simulink model "MPC_Guido_v1_2020a"  (R2020a)
settings: Solver=FixedStepAuto  StartTime=0.0  StopTime=21  RelTol=1e-3
undefined symbols (not defined in the file): Bvx, Bvy, Bw, C, Cvx, Cvy, Cw, D, d, DiscIntNeverNeededParam, Gam, J, K_fsfb, K_int, Kt, l, M, Phi, r, Ti, Ts
libraries: mpclib x3, simulink x1
settings Model: Creator=User  LastModifiedBy=User
settings SolverCC: ZeroCrossControl=EnableAll  ZeroCrossAlgorithm=Adaptive
settings DebuggingCC: IgnoredZcDiagnostic=none

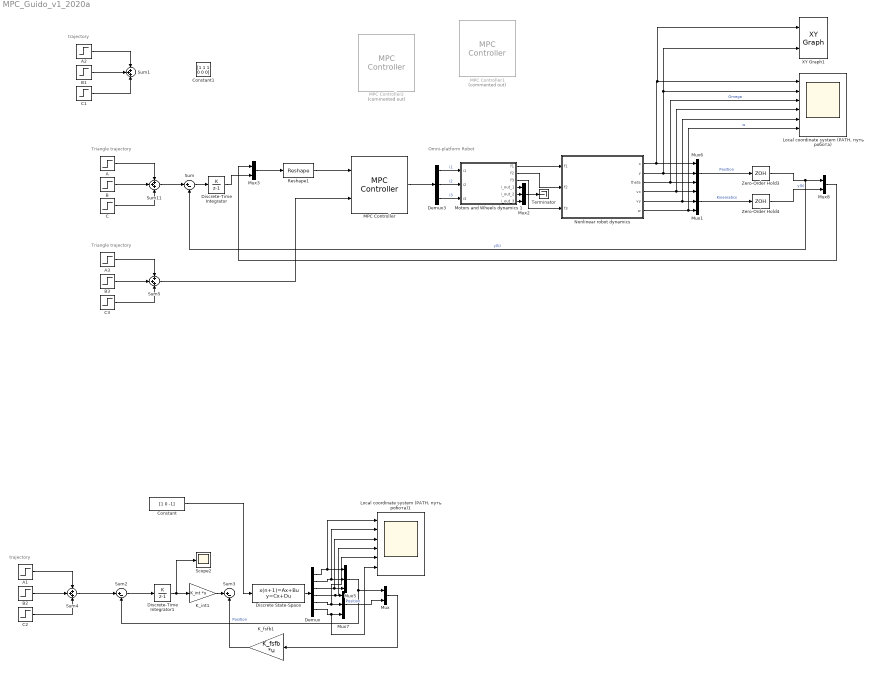
== system MPC_Guido_v1_2020a ==
  note: Omni-platform Robot
  note: Triangle trajectory
  note: trajectory
  note: trajectory
  note: Triangle trajectory
  A : Step  Time=0  Before=[1 0.5 pi/2]  After=[0.5 -sqrt(3)/2 1]  SampleTime=Ts
  A1 : Step  Time=0  Before=[0 0 0]  After=[1 1 0]  SampleTime=Ts
  A2 : Step  Time=0  Before=[0 0 0]  After=[1 1 0]  SampleTime=Ts
  A3 : Step  Time=0  Before=[1 0.5 pi/2 0 0 0 0 0 0]  After=[0.5 -sqrt(3)/2 1 0 0 0 0 0 0]  SampleTime=Ts
  B : Step  Time=7  Before=[0 0 0]  After=[-1 0 1]  SampleTime=Ts
  B1 : Step  Time=6  Before=[0 0 0]  After=[0 0 pi]  SampleTime=Ts
  B2 : Step  Time=6  Before=[0 0 0]  After=[0 0 pi]  SampleTime=Ts
  B3 : Step  Time=7  Before=[0 0 0 0 0 0 0 0 0]  After=[-1 0 1 0 0 0 0 0 0]  SampleTime=Ts
  C : Step  Time=14  Before=[0 0 0]  After=[0.5 sqrt(3)/2 0]  SampleTime=Ts
  C1 : Step  Time=12  Before=[0 0 0]  After=[1 1 0]  SampleTime=Ts
  C2 : Step  Time=12  Before=[0 0 0]  After=[1 1 0]  SampleTime=Ts
  C3 : Step  Time=14  Before=[0 0 0 0 0 0 0 0 0]  After=[0.5 sqrt(3)/2 0 0 0 0 0 0 0]  SampleTime=Ts
  Constant : Constant  Value=[1 0 -1]  SampleTime=Ts
  Constant1 : Constant  Value=[1 1 1 0 0 0]  SampleTime=Ts
  Demux : Demux  Outputs=6
  Demux3 : Demux  Outputs=3
  Discrete State-Space : DiscreteStateSpace  A=Phi  B=Gam  C=C  D=D  SampleTime=Ts
  Discrete-Time Integrator : DiscreteIntegrator  IntegratorMethod=Accumulation: Forward Euler  SampleTime=-1  ICPrevOutput=DiscIntNeverNeededParam  ICPrevScaledInput=DiscIntNeverNeededParam
  Discrete-Time Integrator1 : DiscreteIntegrator  IntegratorMethod=Accumulation: Forward Euler  InitialCondition=[ 0 0 0]  SampleTime=Ts  ICPrevOutput=DiscIntNeverNeededParam  ICPrevScaledInput=DiscIntNeverNeededParam
  K_fsfb1 : Gain  Gain=K_fsfb  Multiplication=Matrix(K*u) (u vector)
  K_int1 : Gain  Gain=K_int  Multiplication=Matrix(K*u) (u vector)
  "Local coordinate system (PATH, путь робота)" : Scope  NumInputPorts=6
  "Local coordinate system (PATH, путь робота)1" : Scope  NumInputPorts=6
  MPC Controller : mpclib/MPC Controller  SCDEnableBlockLinearizationSpecification=on  mpcobj=mpc1  is_multiple=0  enable_value=0  return_u0=off  updateMPCinCallerWorkspace=on  md_inport=off  mv_inport=off  uref_inport=off  return_cost=off  return_mvseq=off  return_qpstatus=off  return_xseq=off  return_state=off  return_ovseq=off  state_inport=off  umin_inport=off  umax_inport=off  ymin_inport=off  ymax_inport=off  cc_inport=off  ywt_inport=off  uwt_inport=off  duwt_inport=off  rhoeps_inport=off  pm_inport=off  MaximumP=10  HorizonChoice=FixedHorizon  n_ts=0.1  n_p=20  n_mv=3  n_md=0  n_ud=0  n_mo=9  n_uo=0  BlockDataType=double  SampleTimeInherited=off  switch_inport=off
  MPC Controller1 : mpclib/MPC Controller  Commented=on  SCDEnableBlockLinearizationSpecification=on  is_multiple=0  enable_value=0  return_u0=off  updateMPCinCallerWorkspace=on  md_inport=off  mv_inport=off  uref_inport=off  return_cost=off  return_mvseq=off  return_qpstatus=off  return_xseq=off  return_state=off  return_ovseq=off  state_inport=off  umin_inport=off  umax_inport=off  ymin_inport=off  ymax_inport=off  cc_inport=off  ywt_inport=off  uwt_inport=off  duwt_inport=off  rhoeps_inport=off  pm_inport=off  MaximumP=10  HorizonChoice=FixedHorizon  n_ts=0.02  n_p=100  n_mv=3  n_md=0  n_ud=0  n_mo=6  n_uo=0  BlockDataType=double  SampleTimeInherited=off  switch_inport=off
  MPC Controller2 : mpclib/MPC Controller  Commented=on  SCDEnableBlockLinearizationSpecification=on  is_multiple=0  enable_value=0  return_u0=off  updateMPCinCallerWorkspace=on  md_inport=off  mv_inport=off  uref_inport=off  return_cost=off  return_mvseq=off  return_qpstatus=off  return_xseq=off  return_state=off  return_ovseq=off  state_inport=off  umin_inport=off  umax_inport=off  ymin_inport=off  ymax_inport=off  cc_inport=off  ywt_inport=off  uwt_inport=off  duwt_inport=off  rhoeps_inport=off  pm_inport=off  MaximumP=10  HorizonChoice=FixedHorizon  n_ts=0.05  n_p=30  n_mv=3  n_md=0  n_ud=0  n_mo=6  n_uo=0  BlockDataType=double  SampleTimeInherited=off  switch_inport=off
  Motors and Wheels dynamics 1 : Subsystem
  Mux : Mux  Inputs=2
  Mux{1..2,5..7} (5 alike) : Mux  Inputs=3
  Mux3 : Mux  Inputs=2
  Mux8 : Mux  Inputs=2
  Nonlinear robot dynamics : Subsystem
  Reshape1 : Reshape  OutputDimensionality=Customize  OutputDimensions=[9,1]
  Scope2 : Scope
  Sum : Sum  Inputs=|+-
  Sum{1,4..5,11} (4 alike) : Sum  Inputs=+++
  Sum2 : Sum  Inputs=|+-
  Sum3 : Sum  Inputs=|+-
  Terminator : Terminator
  XY Graph1 : simulink/Sinks/XY Graph  xmin=-1  xmax=1  ymin=-1  ymax=1  st=-1
  Zero-Order Hold3 : ZeroOrderHold  SampleTime=0.05
  Zero-Order Hold4 : ZeroOrderHold  SampleTime=0.05
  wires:
  Nonlinear robot dynamics/1(x) -> XY Graph1/1, "Local coordinate system (PATH, путь робота)"/1, Mux6/1
  Nonlinear robot dynamics/2(y) -> XY Graph1/2, "Local coordinate system (PATH, путь робота)"/2, Mux6/2
  Nonlinear robot dynamics/3(theta) -> "Local coordinate system (PATH, путь робота)"/3, Mux6/3  "Omega"
  Mux6/1 -> Zero-Order Hold3/1  "Position"
  C/1 -> Sum11/3
  Zero-Order Hold3/1 -> Mux8/1, Sum/2  "y(k)"
  A/1 -> Sum11/1
  B/1 -> Sum11/2
  Nonlinear robot dynamics/5(vy) -> Mux1/2, "Local coordinate system (PATH, путь робота)"/5
  Nonlinear robot dynamics/6(w) -> Mux1/3, "Local coordinate system (PATH, путь робота)"/6  "w"
  Nonlinear robot dynamics/4(vx) -> Mux1/1, "Local coordinate system (PATH, путь робота)"/4
  Demux3/1 -> Motors and Wheels dynamics 1/1(i1)  "i1"
  Demux3/2 -> Motors and Wheels dynamics 1/2(i2)  "i2"
  Demux3/3 -> Motors and Wheels dynamics 1/3(i3)  "i3"
  Zero-Order Hold4/1 -> Mux8/2  "y(k)"
  Mux1/1 -> Zero-Order Hold4/1  "Kinematics"
  C1/1 -> Sum1/3
  A2/1 -> Sum1/1
  B1/1 -> Sum1/2
  K_int1/1 -> Sum3/1
  Sum2/1 -> Discrete-Time Integrator1/1
  Discrete-Time Integrator1/1 -> Scope2/1, K_int1/1
  Discrete State-Space/1 -> Demux/1
  C2/1 -> Sum4/3
  Sum4/1 -> Sum2/1
  A1/1 -> Sum4/1
  B2/1 -> Sum4/2
  Demux/1 -> "Local coordinate system (PATH, путь робота)1"/1, Mux5/1
  Demux/2 -> "Local coordinate system (PATH, путь робота)1"/2, Mux5/2
  Demux/3 -> "Local coordinate system (PATH, путь робота)1"/3, Mux5/3
  Demux/4 -> "Local coordinate system (PATH, путь робота)1"/4, Mux7/1
  Demux/5 -> "Local coordinate system (PATH, путь робота)1"/5, Mux7/2
  Demux/6 -> "Local coordinate system (PATH, путь робота)1"/6, Mux7/3
  Mux5/1 -> Mux/1, Sum2/2  "Position"
  K_fsfb1/1 -> Sum3/2
  Mux7/1 -> Mux/2  "Position"
  Mux/1 -> K_fsfb1/1
  Constant/1 -> Discrete State-Space/1
  Motors and Wheels dynamics 1/1(f1) -> Nonlinear robot dynamics/1(f1)
  Motors and Wheels dynamics 1/2(f2) -> Nonlinear robot dynamics/2(f2)
  Motors and Wheels dynamics 1/3(f3) -> Nonlinear robot dynamics/3(f3)
  Motors and Wheels dynamics 1/4(i_out_1) -> Mux2/1
  Motors and Wheels dynamics 1/5(i_out_2) -> Mux2/2
  Motors and Wheels dynamics 1/6(i_out_3) -> Mux2/3
  Mux2/1 -> Terminator/1
  MPC Controller/1 -> Demux3/1
  Sum/1 -> Discrete-Time Integrator/1
  Sum11/1 -> Sum/1
  Mux3/1 -> Reshape1/1
  Mux8/1 -> Mux3/1
  Reshape1/1 -> MPC Controller/1
  Discrete-Time Integrator/1 -> Mux3/2
  Sum5/1 -> MPC Controller/2
  B3/1 -> Sum5/2
  A3/1 -> Sum5/1
  C3/1 -> Sum5/3

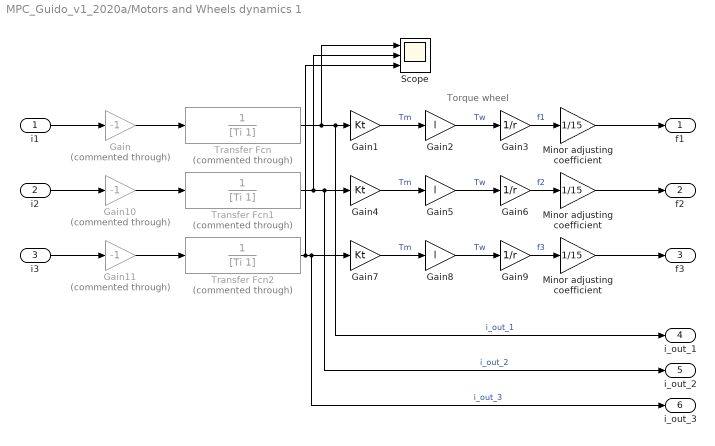
== system MPC_Guido_v1_2020a/Motors and Wheels dynamics 1 ==
  note: Torque wheel
  i1 : Inport
  i2 : Inport  Port=2
  i3 : Inport  Port=3
  Gain : Gain  Commented=through  Gain=-1
  Gain1 : Gain  Gain=Kt
  Gain10 : Gain  Commented=through  Gain=-1
  Gain11 : Gain  Commented=through  Gain=-1
  Gain2 : Gain  Gain=l
  Gain3 : Gain  Gain=1/r
  Gain4 : Gain  Gain=Kt
  Gain5 : Gain  Gain=l
  Gain6 : Gain  Gain=1/r
  Gain7 : Gain  Gain=Kt
  Gain8 : Gain  Gain=l
  Gain9 : Gain  Gain=1/r
  "Minor adjusting coefficient  " : Gain  Gain=1/15
  "Minor adjusting coefficient   " : Gain  Gain=1/15
  "Minor adjusting coefficient    " : Gain  Gain=1/15
  Scope : Scope  NumInputPorts=3
  Transfer Fcn : TransferFcn  Commented=through  Denominator=[Ti 1]  ContinuousStateAttributes='i_out_1'
  Transfer Fcn1 : TransferFcn  Commented=through  Denominator=[Ti 1]  ContinuousStateAttributes='i_out_2'
  Transfer Fcn2 : TransferFcn  Commented=through  Denominator=[Ti 1]  ContinuousStateAttributes='i_out_3'
  f1 : Outport
  f2 : Outport  Port=2
  f3 : Outport  Port=3
  i_out_1 : Outport  Port=4
  i_out_2 : Outport  Port=5
  i_out_3 : Outport  Port=6
  wires:
  i2/1 -> Gain10/1
  Gain1/1 -> Gain2/1  "Tm"
  Gain8/1 -> Gain9/1  "Tw"
  Gain5/1 -> Gain6/1  "Tw"
  Transfer Fcn/1 -> Scope/1, i_out_1/1, Gain1/1  "i_out_1"
  Transfer Fcn2/1 -> Scope/3, i_out_3/1, Gain7/1  "i_out_3"
  i3/1 -> Gain11/1
  Gain2/1 -> Gain3/1  "Tw"
  Gain7/1 -> Gain8/1  "Tm"
  Transfer Fcn1/1 -> Scope/2, i_out_2/1, Gain4/1  "i_out_2"
  Gain4/1 -> Gain5/1  "Tm"
  Gain3/1 -> "Minor adjusting coefficient  "/1  "f1"
  Gain6/1 -> "Minor adjusting coefficient   "/1  "f2"
  i1/1 -> Gain/1
  Gain9/1 -> "Minor adjusting coefficient    "/1  "f3"
  Gain/1 -> Transfer Fcn/1
  Gain10/1 -> Transfer Fcn1/1
  Gain11/1 -> Transfer Fcn2/1
  "Minor adjusting coefficient  "/1 -> f1/1
  "Minor adjusting coefficient   "/1 -> f2/1
  "Minor adjusting coefficient    "/1 -> f3/1

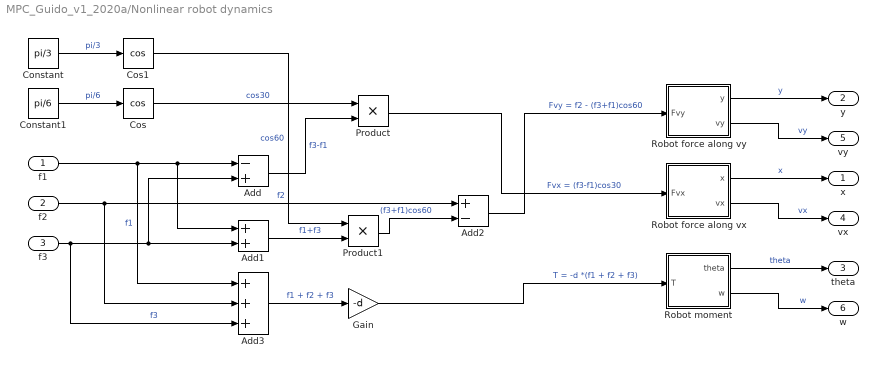
== system MPC_Guido_v1_2020a/Nonlinear robot dynamics ==
  f1 : Inport
  f2 : Inport  Port=2
  f3 : Inport  Port=3
  Add : Sum  Inputs=-+
  Add1 : Sum
  Add2 : Sum  Inputs=+-
  Add3 : Sum  Inputs=+++
  Constant : Constant  Value=pi/3
  Constant1 : Constant  Value=pi/6
  Cos : Trigonometry  Operator=cos
  Cos1 : Trigonometry  Operator=cos
  Gain : Gain  Gain=-d
  Product : Product
  Product1 : Product
  Robot force along vx : Subsystem
  Robot force along vy : Subsystem
  Robot moment : Subsystem
  x : Outport
  y : Outport  Port=2
  theta : Outport  Port=3
  vx : Outport  Port=4
  vy : Outport  Port=5
  w : Outport  Port=6
  wires:
  f3/1 -> Add3/3, Add1/2, Add/2  "f3"
  f1/1 -> Add3/1, Add/1, Add1/1  "f1"
  f2/1 -> Add3/2, Add2/1  "f2"
  Robot force along vy/1(y) -> y/1  "y"
  Robot moment/1(theta) -> theta/1  "theta"
  Robot force along vx/2(vx) -> vx/1  "vx"
  Robot force along vx/1(x) -> x/1  "x"
  Robot moment/2(w) -> w/1  "w"
  Robot force along vy/2(vy) -> vy/1  "vy"
  Add/1 -> Product/2  "f3-f1"
  Constant1/1 -> Cos/1  "pi/6"
  Cos/1 -> Product/1  "cos30"
  Product/1 -> Robot force along vx/1(Fvx)  "Fvx = (f3-f1)cos30"
  Constant/1 -> Cos1/1  "pi/3"
  Cos1/1 -> Product1/1  "cos60"
  Add1/1 -> Product1/2  "f1+f3"
  Product1/1 -> Add2/2  "(f3+f1)cos60"
  Add2/1 -> Robot force along vy/1(Fvy)  "Fvy = f2 - (f3+f1)cos60"
  Add3/1 -> Gain/1  "f1 + f2 + f3"
  Gain/1 -> Robot moment/1(T)  "T = -d *(f1 + f2 + f3)"

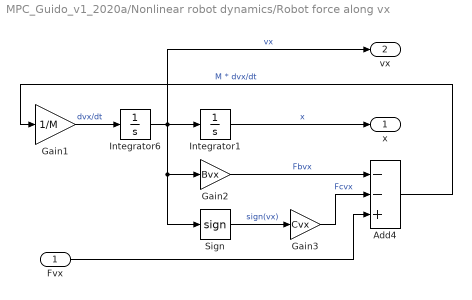
== system MPC_Guido_v1_2020a/Nonlinear robot dynamics/Robot force along vx ==
  Fvx : Inport
  Add4 : Sum  Inputs=--+
  Gain1 : Gain  Gain=1/M
  Gain2 : Gain  Gain=Bvx
  Gain3 : Gain  Gain=Cvx
  Integrator1 : Integrator  ContinuousStateAttributes='x'
  Integrator6 : Integrator  ContinuousStateAttributes='vx'
  Sign : Signum
  x : Outport
  vx : Outport  Port=2
  wires:
  Fvx/1 -> Add4/3
  Sign/1 -> Gain3/1  "sign(vx)"
  Gain2/1 -> Add4/1  "Fbvx"
  Gain3/1 -> Add4/2  "Fcvx"
  Integrator1/1 -> x/1  "x"
  Integrator6/1 -> vx/1, Integrator1/1, Sign/1, Gain2/1  "vx"
  Gain1/1 -> Integrator6/1  "dvx/dt"
  Add4/1 -> Gain1/1  "M * dvx/dt"

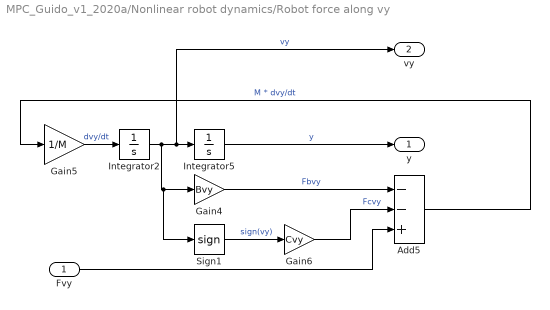
== system MPC_Guido_v1_2020a/Nonlinear robot dynamics/Robot force along vy ==
  Fvy : Inport
  Add5 : Sum  Inputs=--+
  Gain4 : Gain  Gain=Bvy
  Gain5 : Gain  Gain=1/M
  Gain6 : Gain  Gain=Cvy
  Integrator2 : Integrator  ContinuousStateAttributes='vy'
  Integrator5 : Integrator  ContinuousStateAttributes='y'
  Sign1 : Signum
  y : Outport
  vy : Outport  Port=2
  wires:
  Gain5/1 -> Integrator2/1  "dvy/dt"
  Integrator2/1 -> vy/1, Integrator5/1, Sign1/1, Gain4/1  "vy"
  Gain6/1 -> Add5/2  "Fcvy"
  Fvy/1 -> Add5/3
  Add5/1 -> Gain5/1  "M * dvy/dt"
  Sign1/1 -> Gain6/1  "sign(vy)"
  Gain4/1 -> Add5/1  "Fbvy"
  Integrator5/1 -> y/1  "y"

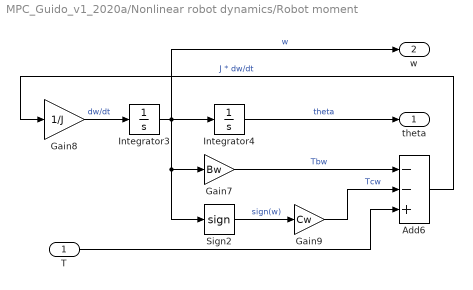
== system MPC_Guido_v1_2020a/Nonlinear robot dynamics/Robot moment ==
  T : Inport
  Add6 : Sum  Inputs=--+
  Gain7 : Gain  Gain=Bw
  Gain8 : Gain  Gain=1/J
  Gain9 : Gain  Gain=Cw
  Integrator3 : Integrator  ContinuousStateAttributes='w'
  Integrator4 : Integrator  ContinuousStateAttributes='theta'
  Sign2 : Signum
  theta : Outport
  w : Outport  Port=2
  wires:
  Integrator3/1 -> w/1, Integrator4/1, Sign2/1, Gain7/1  "w"
  Gain8/1 -> Integrator3/1  "dw/dt"
  Add6/1 -> Gain8/1  "J * dw/dt"
  Gain9/1 -> Add6/2  "Tcw"
  Gain7/1 -> Add6/1  "Tbw"
  Sign2/1 -> Gain9/1  "sign(w)"
  Integrator4/1 -> theta/1  "theta"
  T/1 -> Add6/3
